simulink model "lab1"  (R2023a)
settings: Solver=VariableStepAuto  StartTime=0.0  StopTime=10.0  RelTol=1e-3
values from neighbouring files (symbols this model uses):
  Cm = 1.3    [lab1.m]
  J = 7 * 10^-6    (= 7e-06)    [lab1.m]
  Lia = 0.0015    [lab1.m]
  Lob = 0.013    [lab1.m]
  Ria = 8    [lab1.m]
settings Model: Creator=gbogu  LastModifiedBy=gbogu

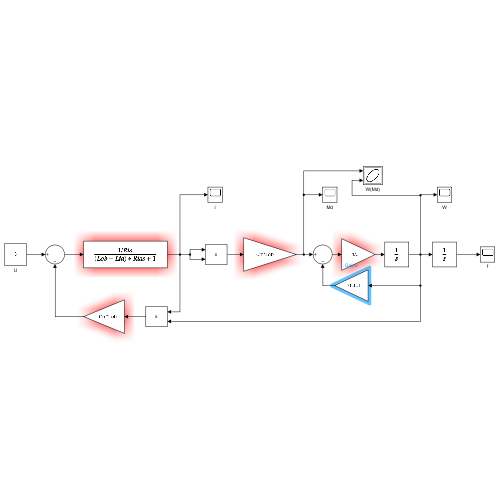
[thumbnail: Simulink's stored preview of the top-level diagram]
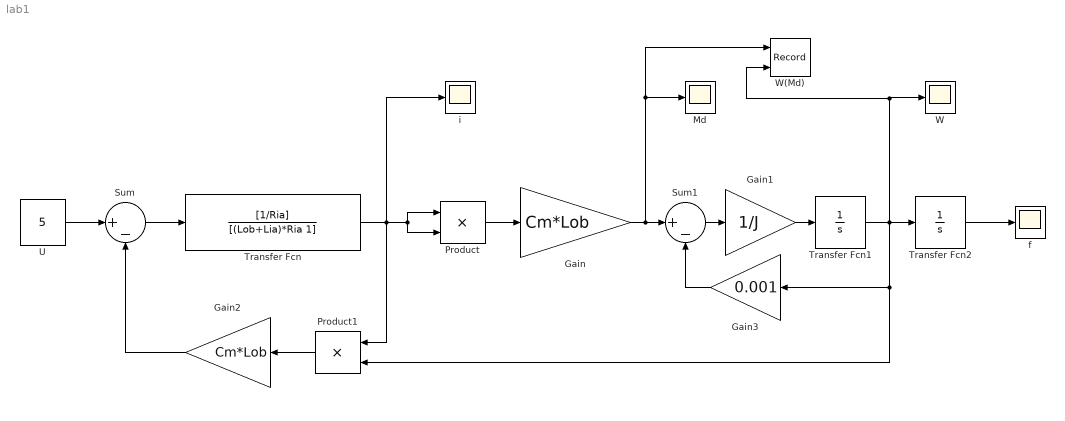
== system lab1 ==
  Gain : Gain  Gain=Cm*Lob
  Gain1 : Gain  Gain=1/J
  Gain2 : Gain  Gain=Cm*Lob
  Gain3 : Gain  Gain=0.001
  Md : Scope
  Product : Product  Inputs=**
  Product1 : Product  Inputs=**
  Sum : Sum  Inputs=|+-
  Sum1 : Sum  Inputs=|+-
  Transfer Fcn : TransferFcn  Numerator=[1/Ria]  Denominator=[(Lob+Lia)*Ria 1]
  Transfer Fcn1 : TransferFcn  Denominator=[1 0]
  Transfer Fcn2 : TransferFcn  Denominator=[1 0]
  U : Constant  Value=5
  W : Scope
  W(Md) : Record  FileSettingsInternal="{\"entries\":[{\"content\":{\"excelSettings\":{\"content\":{},\"type\":\"Streamout.ExcelSettings\"}},\"type\":\"Streamout.FileSettingStorage\",\"uuid\":\"261da392-665f-4892-a6d2-942edc7b2c74\"}],\"packageUris\":[\"http://schema.mathworks.com/mf0/streamout_blocks/R2020a\"],\"version\":\"1.0\"}"  Layout=[1 1]  SignalsInternal="{\"entries\":[{\"content\":{\"signals\":[{\"content\":{\"blockPath\":[\"lab1/W(Md)\"],\"dimensions\":[1],\"domain\":\"lab1/W(Md)\",\"lineColor\":\"#a2142f\",\"plots\":[1],\"port\":1,\"signalID\":8,\"signalName\":\"Gain\"},\"type\":\"RecordBlkView.Signal\",\"uuid\":\"5bea3d3c-ec2e-4009-9e5c-529c4175c7c0\"},{\"content\":{\"blockPath\":[\"lab1/W(Md)\"],\"dimensions\":[1],\"domain\":\"lab1/W(Md)\",\"lineColor\":\"#139fff\",\"plots\":[1],\"port\":2,\"signalID\":11,\"signalName\":\"Transfer Fcn1\"},\"type\":\"RecordBlkView.Signal\",\"uuid\":\"25d2efb7-f2a6-494b-8681-c9f4c4926a2b\"}]},\"type\":\"RecordBlkView.InputSignals\",\"uuid\":\"2647890e-64ab-4654-aa1e-eb37abe5a350\"}],\"packageUris\":[\"http://schema.mathworks.com/mf0/streamout_blocks/R2020a\"],\"version\":\"1.0\"}"  VisualizationBindings="{\"xyplotplugin\":{\"info\":[{\"series\":[{\"bindingParametersList\":[{\"parameter\":\"X-Axis\",\"signalID\":8,\"signalName\":\"Gain\"},{\"parameter\":\"Y-Axis\",\"signalID\":11,\"signalName\":\"Transfer Fcn1\"}],\"seriesID\":25090}],\"subplotID\":1}]}}"  CompatibilityTag=XY
  f : Scope
  i : Scope
  wires:
  Gain1/1 -> Transfer Fcn1/1
  Transfer Fcn2/1 -> f/1
  Gain2/1 -> Sum/2
  Product1/1 -> Gain2/1
  Gain/1 -> Sum1/1, W(Md)/1, Md/1
  Product/1 -> Gain/1
  Transfer Fcn1/1 -> Gain3/1, Product1/2, W(Md)/2, W/1, Transfer Fcn2/1
  Transfer Fcn/1 -> Product1/1, i/1, Product/2, Product/1
  U/1 -> Sum/1
  Sum/1 -> Transfer Fcn/1
  Sum1/1 -> Gain1/1
  Gain3/1 -> Sum1/2
